simulink model "FiltroAcoplador"  (Simulink 7.7)
settings: Solver=ode3  StartTime=0.0  StopTime=0.01  RelTol=1e-3
libraries: commchan3 x2, commsink2 x2, commrandsrc2 x2, dspsigops x2
settings Model: Creator=hp  LastModifiedBy=hp

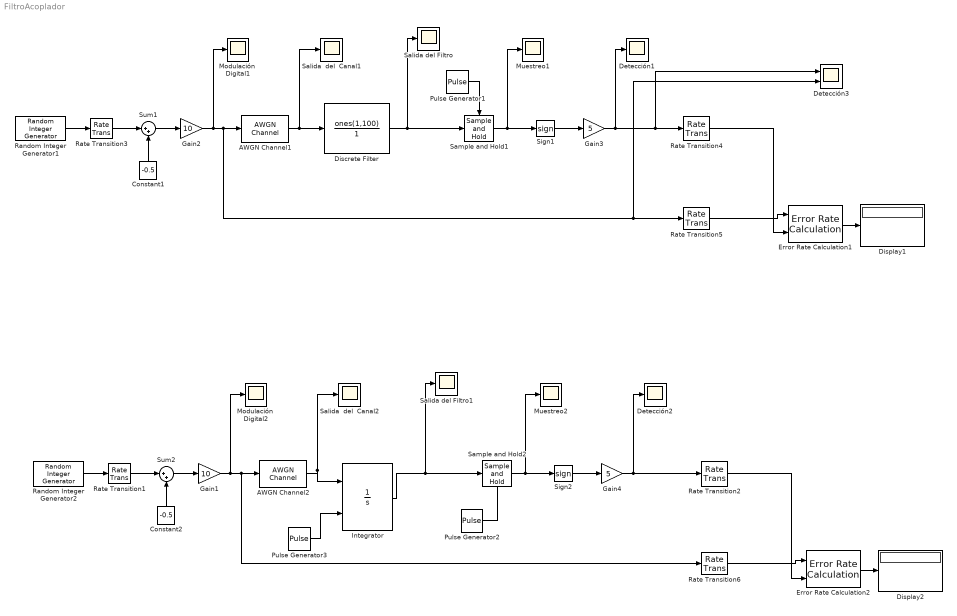
== system FiltroAcoplador ==
  AWGN Channel1 : commchan3/AWGN Channel  SystemSampleTime=-1  InputProcessing=Columns as channels (frame based)  seed=randseed  noiseMode=Variance from mask  EbNodB=10  EsNodB=10  SNRdB=10  bitsPerSym=1  Ps=1  Tsym=1  variance=0
  AWGN Channel2 : commchan3/AWGN Channel  SystemSampleTime=-1  InputProcessing=Columns as channels (frame based)  seed=randseed  noiseMode=Variance from mask  EbNodB=10  EsNodB=10  SNRdB=10  bitsPerSym=1  Ps=1  Tsym=1  variance=0
  Constant1 : Constant  Value=-0.5
  Constant2 : Constant  Value=-0.5
  Detección1 : Scope
      settings: TimeRange=0.09999999999999965  YMin=-6  YMax=6
  Detección2 : Scope
      settings: TimeRange=0.09999999999999965  YMin=-6  YMax=6  SaveName=ScopeData5
  Detección3 : Scope  NumInputPorts=2
      settings: TimeRange=0.01  YMin=-7~-7  YMax=7~7  SaveName=ScopeData10  MaxDataPoints=1000
  Discrete Filter : DiscreteFilter  Numerator=ones(1,100)  Denominator=1  SampleTime=1e-5
  Display1 : Display
  Display2 : Display
  Error Rate Calculation1 : commsink2/Error Rate Calculation  N=1  st_delay=0  cp_mode=Entire frame  subframe=[]  PMode=Port  WsName=ErrorVec  RsMode2=off  stop=off  numErr=100  maxBits=1e6
  Error Rate Calculation2 : commsink2/Error Rate Calculation  N=1  st_delay=0  cp_mode=Entire frame  subframe=[]  PMode=Port  WsName=ErrorVec  RsMode2=off  stop=off  numErr=100  maxBits=1e6
  Gain1 : Gain  Gain=10
  Gain2 : Gain  Gain=10
  Gain3 : Gain  Gain=5
  Gain4 : Gain  Gain=5
  Integrator : Integrator  ExternalReset=rising
  Modulación  Digital1 : Scope
      settings: TimeRange=0.09999999999999965  YMin=-6  YMax=6
  Modulación  Digital2 : Scope
      settings: TimeRange=0.09999999999999965  YMin=-6  YMax=6  SaveName=ScopeData6
  Muestreo1 : Scope
      settings: TimeRange=0.09999999999999965  YMin=-6  YMax=6  SaveName=ScopeData2
  Muestreo2 : Scope
      settings: TimeRange=0.09999999999999965  YMin=-6  YMax=6  SaveName=ScopeData7
  Pulse Generator1 : DiscretePulseGenerator  PulseType=Time based  Period=0.001  PulseWidth=10
  Pulse Generator2 : DiscretePulseGenerator  PulseType=Time based  Period=0.001  PulseWidth=10  PhaseDelay=.99*1e-5
  Pulse Generator3 : DiscretePulseGenerator  PulseType=Time based  Period=0.001  PulseWidth=10
  Random Integer Generator1 : commrandsrc2/Random Integer Generator  SystemSampleTime=-1  mul=2  seed=randseed  Ts=0.001  frameBased=off  sampPerFrame=1  orient=off  outDataType=double
  Random Integer Generator2 : commrandsrc2/Random Integer Generator  SystemSampleTime=-1  mul=2  seed=randseed  Ts=0.001  frameBased=off  sampPerFrame=1  orient=off  outDataType=double
  Rate Transition1 : RateTransition  OutPortSampleTime=0.00002
  Rate Transition{2,4..6} (4 alike) : RateTransition  OutPortSampleTime=0.001
  Rate Transition3 : RateTransition  OutPortSampleTime=1e-5
  Salida del Filtro : Scope
      settings: TimeRange=0.09999999999999965  YMin=-6  YMax=6  SaveName=ScopeData3
  Salida del Filtro1 : Scope
      settings: TimeRange=0.09999999999999965  YMin=-6  YMax=6  SaveName=ScopeData8
  Salida  del  Canal1 : Scope
      settings: TimeRange=0.09999999999999965  YMin=-6  YMax=6  SaveName=ScopeData4
  Salida  del  Canal2 : Scope
      settings: TimeRange=0.09999999999999965  YMin=-6  YMax=6  SaveName=ScopeData9
  Sample and Hold1 : dspsigops/Sample and Hold  SystemSampleTime=-1  trig=Rising edge  initCond=0  latchinput=off
  Sample and Hold2 : dspsigops/Sample and Hold  SystemSampleTime=-1  trig=Rising edge  initCond=0  latchinput=off
  Sign1 : Signum
  Sign2 : Signum
  Sum1 : Sum  Inputs=|++
  Sum2 : Sum  Inputs=|++
  wires:
  Random Integer Generator1/1 -> Rate Transition3/1
  Rate Transition3/1 -> Sum1/1
  Constant1/1 -> Sum1/2
  Sum1/1 -> Gain2/1
  Gain2/1 -> Modulación  Digital1/1, AWGN Channel1/1, Rate Transition5/1, Detección3/2
  AWGN Channel1/1 -> Salida  del  Canal1/1, Discrete Filter/1
  Pulse Generator1/1 -> Sample and Hold1/Trigger
  Sample and Hold1/1 -> Sign1/1, Muestreo1/1
  Sign1/1 -> Gain3/1
  Gain3/1 -> Detección1/1, Rate Transition4/1, Detección3/1
  Rate Transition5/1 -> Error Rate Calculation1/1
  Rate Transition4/1 -> Error Rate Calculation1/2
  Error Rate Calculation1/1 -> Display1/1
  Discrete Filter/1 -> Sample and Hold1/1, Salida del Filtro/1
  Random Integer Generator2/1 -> Rate Transition1/1
  Rate Transition1/1 -> Sum2/1
  Constant2/1 -> Sum2/2
  Sum2/1 -> Gain1/1
  Gain1/1 -> Modulación  Digital2/1, AWGN Channel2/1, Rate Transition6/1
  AWGN Channel2/1 -> Salida  del  Canal2/1, Integrator/1
  Sample and Hold2/1 -> Sign2/1, Muestreo2/1
  Sign2/1 -> Gain4/1
  Gain4/1 -> Detección2/1, Rate Transition2/1
  Rate Transition6/1 -> Error Rate Calculation2/1
  Rate Transition2/1 -> Error Rate Calculation2/2
  Error Rate Calculation2/1 -> Display2/1
  Integrator/1 -> Sample and Hold2/1, Salida del Filtro1/1
  Pulse Generator3/1 -> Integrator/2
  Pulse Generator2/1 -> Sample and Hold2/Trigger
